simulink model "RendezvousSimulator"  (R2026a)
settings: Solver=ode4  StopTime=7200  FixedStep=0.01
values from neighbouring files (symbols this model uses):
  beta_in = zeros(3,1)    [std_run_docking.m]    (also in std_run_rendezvous.m)
  dt = 0.01    [std_run_docking.m]    (also in std_run_rendezvous.m)
  K = lqr(A,B,Q, R)    [std_run_rendezvous.m]
  muEarth = 3.986004418e14    (= 398600441800000)    [std_run_docking.m]    (also in std_run_rendezvous.m)
  P_in = eye(6) * 1e-4    [std_run_docking.m]    (also in std_run_rendezvous.m)
  q_ic = [1;0;0;0]    [std_run_docking.m]    (also in std_run_rendezvous.m)
  u_ref = -B\(A*xref)    [std_run_rendezvous.m]
  xref = [chaser_CoM_target; 0; 0; 0]    [std_run_docking.m]    (also in std_run_rendezvous.m = [-250, 0, 0, 0.05, 0, 0]')
undefined symbols (not defined in the file or in its folder): ADCS, chaser, control, RCS, RW, target
libraries: aerolibutil x6, simulink x5, simulink_extras x3, matrix_library x1, vrlib x1, mpclib x1, aerolibnav x1
settings Model: SimulationMode=accelerator  Creator=Guilherme  LastModifiedBy=User

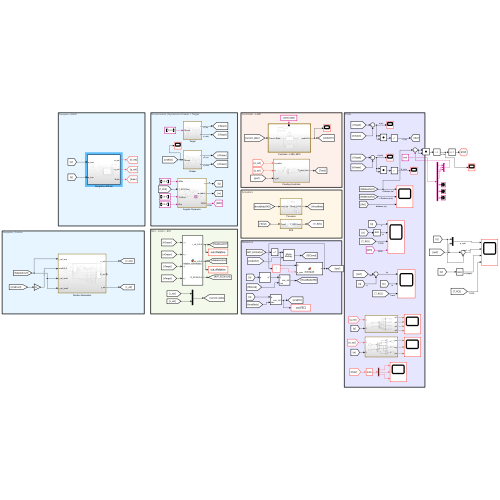
[thumbnail: Simulink's stored preview of the top-level diagram]
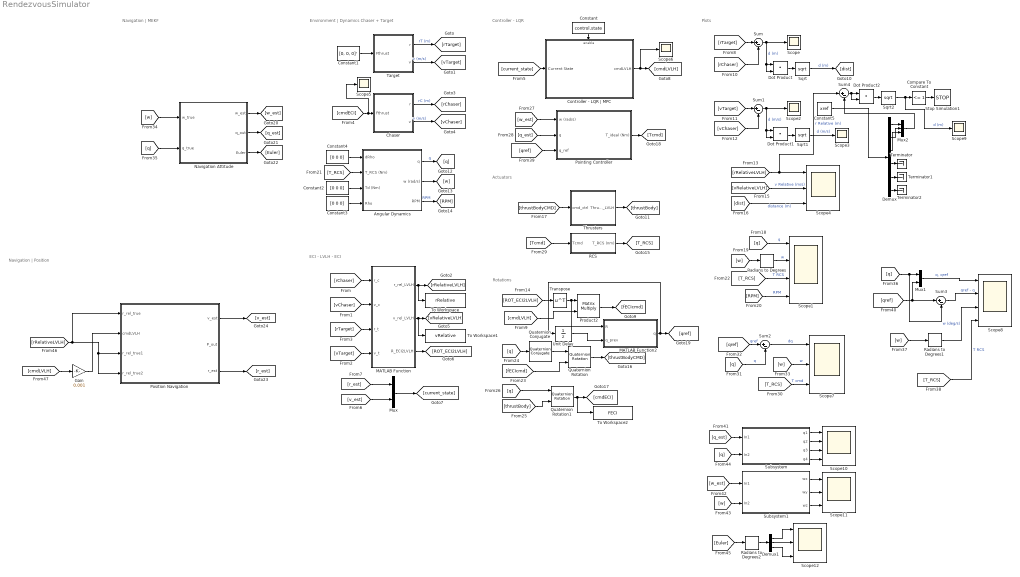
== system RendezvousSimulator ==
  note: Rotations
  note: Actuators
  note: ECI - LVLH - ECI
  note: Controller - LQR
  note: Environment | Dynamics Chaser + Target
  note: Navigation | MEKF
  note: Plots
  note: Navigation | Position
  Angular Dynamics : Subsystem
  Chaser : Subsystem
  Compare To Constant : simulink/Logic and Bit Operations/Compare To Constant  relop=<=  const=1  OutDataTypeStr=boolean
  Constant : Constant  Value=control.state
  Constant1 : Constant  Value=[0, 0, 0]'
  Constant2 : Constant  Value=[0 0 0]
  Constant3 : Constant  Value=[0 0 0]
  Constant4 : Constant  Value=[0 0 0]
  Constant5 : Constant  Value=xref
  Controller - LQR | MPC : Subsystem
  Demux : Demux  Outputs=6
  Demux1 : Demux  Outputs=3
  Dot Product : DotProduct  OutDataTypeStr=Inherit: Inherit via internal rule
  Dot Product1 : DotProduct  OutDataTypeStr=Inherit: Inherit via internal rule
  Dot Product2 : DotProduct  OutDataTypeStr=Inherit: Inherit via internal rule
  Gain : Gain  Gain=0.001
  MATLAB Function : MATLAB Function  TreatAsAtomicUnit=on
  MATLAB Function2 : MATLAB Function  TreatAsAtomicUnit=on
  Mux : Mux  Inputs=2
  Mux1 : Mux  Inputs=2
  Mux2 : Mux  Inputs=3
  Navigation Attitude : Subsystem
  Pointing Controller : Subsystem
  Position Navigation : Subsystem
  Product2 : Product  Multiplication=Matrix(*)
  Quaternion Conjugate : aerolibutil/Quaternion Conjugate
  Quaternion Rotation : aerolibutil/Quaternion Rotation
  Quaternion Rotation1 : aerolibutil/Quaternion Rotation
  RCS : Subsystem
  Radians to Degrees : simulink_extras/Transformations/Radians to Degrees
  Radians to Degrees1 : simulink_extras/Transformations/Radians to Degrees
  Radians to Degrees2 : simulink_extras/Transformations/Radians to Degrees
  Scope{,2..3,5..6,9} (6 alike) : Scope
      Scope settings: ActiveDisplayYMinimum=-1060.8843099508601  ActiveDisplayYMaximum=894.14977464646563
      Scope2 settings: ActiveDisplayYMinimum=-1  ActiveDisplayYMaximum=1  DataLoggingVariableName=ScopeData2
      Scope3 settings: ActiveDisplayYMinimum=-1  ActiveDisplayYMaximum=1  DataLoggingVariableName=ScopeData3
      Scope5 settings: ActiveDisplayYMinimum=-8.2979644162863622  ActiveDisplayYMaximum=33.856564576377387  DataLoggingVariableName=ScopeData5
      Scope6 settings: ActiveDisplayYMinimum=-1  ActiveDisplayYMaximum=1  DataLoggingVariableName=ScopeData6
      Scope9 settings: ActiveDisplayYMinimum=-855.71515275184811  ActiveDisplayYMaximum=7759.3343036097422  DataLoggingVariableName=ScopeData16
  Scope1 : Scope  NumInputPorts=4
      settings: ActiveDisplayYMinimum=-0.12499999999999997  ActiveDisplayYMaximum=1.125  DataLoggingVariableName=ScopeData7
  Scope10 : Scope  NumInputPorts=4
      settings: ActiveDisplayYMinimum=-1  ActiveDisplayYMaximum=1  DataLoggingVariableName=ScopeData17
  Scope{4,7,11..12} (4 alike) : Scope  NumInputPorts=3
      Scope11 settings: ActiveDisplayYMinimum=-0.006211242993111819  ActiveDisplayYMaximum=0.0063918392422366421  DataLoggingVariableName=ScopeData18
      Scope12 settings: ActiveDisplayYMinimum=-0.04294458122283102  ActiveDisplayYMaximum=0.042529284958808582  DataLoggingVariableName=ScopeData19
      Scope4 settings: ActiveDisplayYMinimum=-521.32635380799536  ActiveDisplayYMaximum=173.1359744426077  DataLoggingVariableName=ScopeData4
      Scope7 settings: ActiveDisplayYMinimum=-0.011828379058664178  ActiveDisplayYMaximum=0.0155264540868424  DataLoggingVariableName=ScopeData8
  Scope8 : Scope  NumInputPorts=4
      settings: ActiveDisplayYMinimum=-1.130569243154838  ActiveDisplayYMaximum=1.2367299159060932  DataLoggingVariableName=ScopeData12
  Sqrt : Sqrt
  Sqrt1 : Sqrt
  Sqrt2 : Sqrt
  Stop Simulation1 : Stop
  Subsystem : Subsystem
  Subsystem1 : Subsystem
  Sum{,1..4} (5 alike) : Sum  Inputs=|+-
  Target : Subsystem
  Terminator : Terminator
  Terminator1 : Terminator
  Terminator2 : Terminator
  Thrusters : Subsystem
  To Workspace : ToWorkspace  VariableName=rRelative  SaveFormat=Structure With Time  SampleTime=-1
  To Workspace1 : ToWorkspace  VariableName=vRelative  SaveFormat=Structure With Time  SampleTime=-1
  To Workspace2 : ToWorkspace  VariableName=FECI  SaveFormat=Structure With Time  SampleTime=-1
  Transpose : Math  Operator=transpose
  Unit Delay : UnitDelay  InitialCondition=[1;0;0;0]  SampleTime=dt
  wires:
  Constant1/1 -> Target/1(Fthrust)
  Target/1(r) -> [rTarget]  "rT (m)"
  Target/2(v) -> [vTarget]  "v (m/s)"
  Chaser/1(r) -> [rChaser]  "rC (m)"
  Chaser/2(v) -> [vChaser]  "v (m/s)"
  Mux/1 -> [current_state]
  [r_est] -> Mux/1
  [v_est] -> Mux/2
  Transpose/1 -> MATLAB Function2/1(R), Product2/1
  [ROT_ECI2LVLH] -> Transpose/1
  [cmdLVLH] -> Product2/2
  [cmdECI] -> Scope5/1, Chaser/1(Fthrust)
  [rChaser] -> MATLAB Function/1(r_c)
  [vChaser] -> MATLAB Function/2(v_c)
  [vTarget] -> MATLAB Function/4(v_t)
  [rTarget] -> MATLAB Function/3(r_t)
  MATLAB Function/1(r_rel_LVLH) -> [rRelativeLVLH], To Workspace/1
  MATLAB Function/2(v_rel_LVLH) -> [vRelativeLVLH], To Workspace1/1
  MATLAB Function/3(R_ECI2LVLH) -> [ROT_ECI2LVLH]
  Product2/1 -> [fECIcmd]
  [current_state] -> Controller - LQR | MPC/1(Current State)
  Controller - LQR | MPC/1(cmdLVLH) -> Scope6/1, [cmdLVLH]
  [rTarget] -> Sum/1
  [rChaser] -> Sum/2
  Sum/1 -> Scope/1, Dot Product/2, Dot Product/1  "d (m)"
  Dot Product/1 -> Sqrt/1
  Sqrt/1 -> [dist]  "d (m)"
  Sqrt1/1 -> Scope3/1  "d (m/s)"
  Sum1/1 -> Scope2/1, Dot Product1/2, Dot Product1/1  "d (m/s)"
  Dot Product1/1 -> Sqrt1/1
  [vChaser] -> Sum1/2
  [vTarget] -> Sum1/1
  Compare To Constant/1 -> Stop Simulation1/1
  [rRelativeLVLH] -> Sum4/1, Scope4/1  "r Relative (m)"
  [vRelativeLVLH] -> Scope4/2  "v Relative (m/s)"
  [dist] -> Scope4/3  "distance (m)"
  [thrustBodyCMD] -> Thrusters/1(cmd_ctrl)
  Thrusters/1(Thrust_LVLH) -> [thrustBody]
  Constant/1 -> Controller - LQR | MPC/Enable
  Constant2/1 -> Angular Dynamics/3(Td (Nm))
  Constant3/1 -> Angular Dynamics/4(Rho)
  Constant4/1 -> Angular Dynamics/1(dRho)
  Angular Dynamics/1(q) -> [q]  "q"
  Angular Dynamics/2(w (rad/s)) -> [w]
  Angular Dynamics/3(RPM) -> [RPM]  "RPM"
  [q] -> Scope1/1  "q"
  Radians to Degrees/1 -> Scope1/2  "w"
  [w] -> Radians to Degrees/1
  [RPM] -> Scope1/4  "RPM"
  [Tcmd] -> RCS/1(Tcmd)
  RCS/1(T_RCS (nm)) -> [T_RCS]
  [T_RCS] -> Scope1/3  "T RCS"
  [q] -> Quaternion Conjugate/1
  Quaternion Conjugate/1 -> Quaternion Rotation/1
  [fECIcmd] -> Quaternion Rotation/2
  Quaternion Rotation/1 -> [thrustBodyCMD]
  [thrustBody] -> Quaternion Rotation1/2
  [q] -> Quaternion Rotation1/1
  Quaternion Rotation1/1 -> To Workspace2/1, [cmdECI]
  [w_est] -> Pointing Controller/1(w (rad/s))
  [q_est] -> Pointing Controller/2(q)
  Pointing Controller/1(T_ideal (Nm)) -> [Tcmd]
  MATLAB Function2/1(q) -> Unit Delay/1, [qref]
  [qref] -> Pointing Controller/3(q_ref)
  [w] -> Scope7/2  "w"
  Sum2/1 -> Scope7/1  "dq"
  [q] -> Sum2/2  "q"
  [qref] -> Sum2/1  "qref"
  [T_RCS] -> Scope7/3  "T cmd"
  [q] -> Sum3/2, Mux1/1
  [qref] -> Sum3/1, Mux1/2
  Mux1/1 -> Scope8/1  "q, qref"
  Sum3/1 -> Scope8/2  "qref - q"
  [w] -> Radians to Degrees1/1
  Radians to Degrees1/1 -> Scope8/3  "w (deg/s)"
  [T_RCS] -> Angular Dynamics/2(T_RCS (Nm))
  [T_RCS] -> Scope8/4  "T RCS"
  Sum4/1 -> Dot Product2/2, Dot Product2/1
  Dot Product2/1 -> Sqrt2/1
  Sqrt2/1 -> Scope9/1, Compare To Constant/1  "d (m)"
  Demux/1 -> Mux2/1
  Demux/2 -> Mux2/2
  Demux/3 -> Mux2/3
  Constant5/1 -> Demux/1
  Mux2/1 -> Sum4/2
  Demux/4 -> Terminator/1
  Demux/5 -> Terminator1/1
  Demux/6 -> Terminator2/1
  [w] -> Navigation Attitude/1(w_true)
  [q] -> Navigation Attitude/2(q_true)
  Navigation Attitude/1(w_est) -> [w_est]
  Navigation Attitude/2(q_out) -> [q_est]
  Navigation Attitude/3(Euler) -> [Euler]
  [Euler] -> Radians to Degrees2/1
  Radians to Degrees2/1 -> Demux1/1
  Demux1/1 -> Scope12/1
  Demux1/2 -> Scope12/2
  Demux1/3 -> Scope12/3
  [q_est] -> Subsystem/1(In1)
  [q] -> Subsystem/2(In2)
  Subsystem/1(q1) -> Scope10/1
  Subsystem/2(q2) -> Scope10/2
  Subsystem/3(q3) -> Scope10/3
  Subsystem/4(q4) -> Scope10/4
  [w] -> Subsystem1/2(In2)
  Subsystem1/1(wx) -> Scope11/1
  Subsystem1/2(wy) -> Scope11/2
  Subsystem1/3(wz) -> Scope11/3
  [w_est] -> Subsystem1/1(In1)
  Unit Delay/1 -> MATLAB Function2/2(q_prev)
  Position Navigation/3(r_est) -> [r_est]
  Gain/1 -> Position Navigation/2(cmdLVLH)
  [cmdLVLH] -> Gain/1
  Position Navigation/1(v_est) -> [v_est]
  [rRelativeLVLH] -> Position Navigation/4(r_rel_true2), Position Navigation/3(r_rel_true1), Position Navigation/1(r_rel_true)

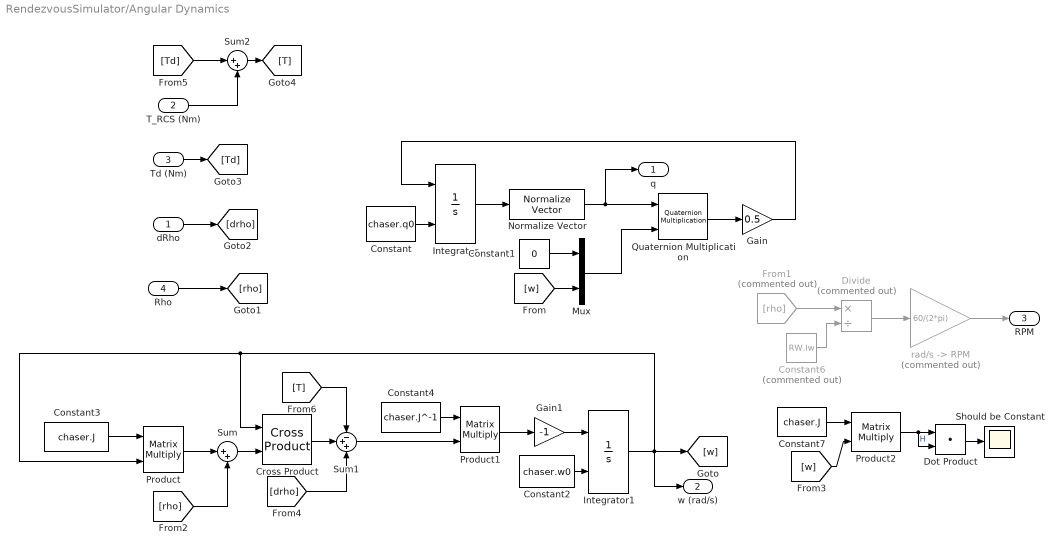
== system RendezvousSimulator/Angular Dynamics ==
  dRho : Inport
  T_RCS (Nm) : Inport  Port=2
  Td (Nm) : Inport  Port=3
  Rho : Inport  Port=4
  Constant : Constant  Value=chaser.q0
  Constant1 : Constant  Value=0
  Constant2 : Constant  Value=chaser.w0
  Constant3 : Constant  Value=chaser.J
  Constant4 : Constant  Value=chaser.J^-1
  Constant6 : Constant  Commented=on  Value=RW.Iw
  Constant7 : Constant  Value=chaser.J
  Cross Product : matrix_library/Cross Product
  Divide : Product  Commented=on  Inputs=*/
  Dot Product : DotProduct  OutDataTypeStr=Inherit: Inherit via internal rule
  From1 : From  Commented=on  GotoTag=rho
  Gain : Gain  Gain=0.5
  Gain1 : Gain  Gain=-1
  Integrator : Integrator  InitialConditionSource=external
  Integrator1 : Integrator  InitialConditionSource=external
  Mux : Mux  Inputs=2
  Normalize Vector : vrlib/Utilities/Normalize Vector  maxzero=0
  Product : Product  Multiplication=Matrix(*)
  Product1 : Product  Multiplication=Matrix(*)
  Product2 : Product  Multiplication=Matrix(*)
  Quaternion Multiplication : aerolibutil/Quaternion Multiplication
  Should be Constant : Scope
      settings: ActiveDisplayYMinimum=4.5666666666666505E-5  ActiveDisplayYMaximum=6.566666666666693E-5
  Sum : Sum  Inputs=|++
  Sum1 : Sum  Inputs=-++
  Sum2 : Sum  Inputs=|++
  "rad/s -> RPM" : Gain  Commented=on  Gain=60/(2*pi)
  q : Outport
  w (rad/s) : Outport  Port=2
  RPM : Outport  Port=3
  wires:
  Normalize Vector/1 -> q/1, Quaternion Multiplication/1
  Quaternion Multiplication/1 -> Gain/1
  Integrator1/1 -> w (rad/s)/1, Product/2, Cross Product/1, [w]
  Constant/1 -> Integrator/2
  Constant2/1 -> Integrator1/2
  [rho] -> Sum/2
  Product1/1 -> Gain1/1
  Gain/1 -> Integrator/1
  Sum/1 -> Cross Product/2
  Constant4/1 -> Product1/1
  Integrator/1 -> Normalize Vector/1
  Sum1/1 -> Product1/2
  Constant1/1 -> Mux/1
  Mux/1 -> Quaternion Multiplication/2
  Product/1 -> Sum/1
  Cross Product/1 -> Sum1/2
  [w] -> Mux/2
  [T] -> Sum1/1
  Gain1/1 -> Integrator1/1
  Constant3/1 -> Product/1
  From1/1 -> Divide/1
  Constant6/1 -> Divide/2
  Divide/1 -> "rad/s -> RPM"/1
  "rad/s -> RPM"/1 -> RPM/1
  Constant7/1 -> Product2/1
  Dot Product/1 -> Should be Constant/1
  Product2/1 -> Dot Product/2, Dot Product/1  "H"
  [w] -> Product2/2
  Td (Nm)/1 -> [Td]
  [Td] -> Sum2/1
  T_RCS (Nm)/1 -> Sum2/2
  Sum2/1 -> [T]
  [drho] -> Sum1/3
  Rho/1 -> [rho]
  dRho/1 -> [drho]

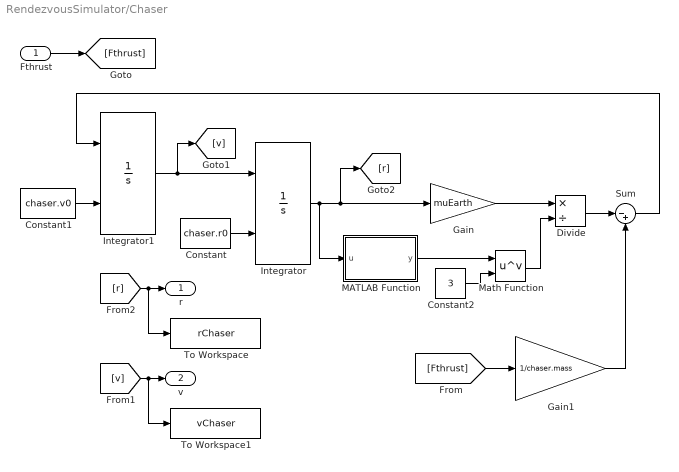
== system RendezvousSimulator/Chaser ==
  Fthrust : Inport
  Constant : Constant  Value=chaser.r0
  Constant1 : Constant  Value=chaser.v0
  Constant2 : Constant  Value=3
  Divide : Product  Inputs=*/
  Gain : Gain  Gain=muEarth
  Gain1 : Gain  Gain=1/chaser.mass
  Integrator : Integrator  InitialConditionSource=external
  Integrator1 : Integrator  InitialConditionSource=external
  MATLAB Function : MATLAB Function  TreatAsAtomicUnit=on
  Math Function : Math  Operator=pow
  Sum : Sum  Inputs=|-+
  To Workspace : ToWorkspace  VariableName=rChaser  SaveFormat=Structure With Time  SampleTime=-1
  To Workspace1 : ToWorkspace  VariableName=vChaser  SaveFormat=Structure With Time  SampleTime=-1
  r : Outport
  v : Outport  Port=2
  wires:
  Integrator/1 -> MATLAB Function/1(u), [r], Gain/1
  Constant1/1 -> Integrator1/2
  Gain/1 -> Divide/1
  Divide/1 -> Sum/1
  Constant/1 -> Integrator/2
  Sum/1 -> Integrator1/1
  Integrator1/1 -> Integrator/1, [v]
  Fthrust/1 -> [Fthrust]
  [Fthrust] -> Gain1/1
  Gain1/1 -> Sum/2
  [v] -> To Workspace1/1, v/1
  [r] -> To Workspace/1, r/1
  MATLAB Function/1(y) -> Math Function/1
  Constant2/1 -> Math Function/2
  Math Function/1 -> Divide/2

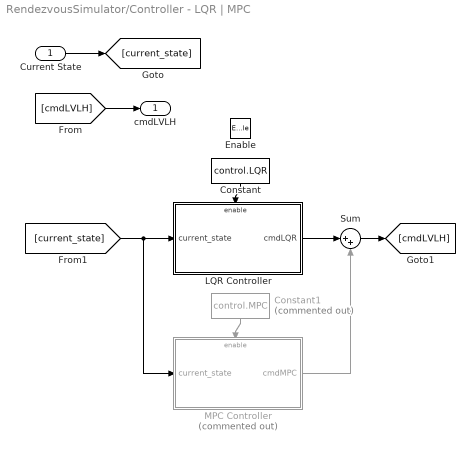
== system RendezvousSimulator/Controller - LQR | MPC ==
  Current State : Inport
  Enable : EnablePort
  Constant : Constant  Value=control.LQR
  Constant1 : Constant  Commented=on  Value=control.MPC
  LQR Controller : Subsystem
  MPC Controller : Subsystem  Commented=on
  Sum : Sum  Inputs=|++
  cmdLVLH : Outport
  wires:
  Current State/1 -> [current_state]
  [cmdLVLH] -> cmdLVLH/1
  Constant/1 -> LQR Controller/Enable
  Constant1/1 -> MPC Controller/Enable
  LQR Controller/1(cmdLQR) -> Sum/1
  MPC Controller/1(cmdMPC) -> Sum/2
  Sum/1 -> [cmdLVLH]
  [current_state] -> MPC Controller/1(current_state), LQR Controller/1(current_state)

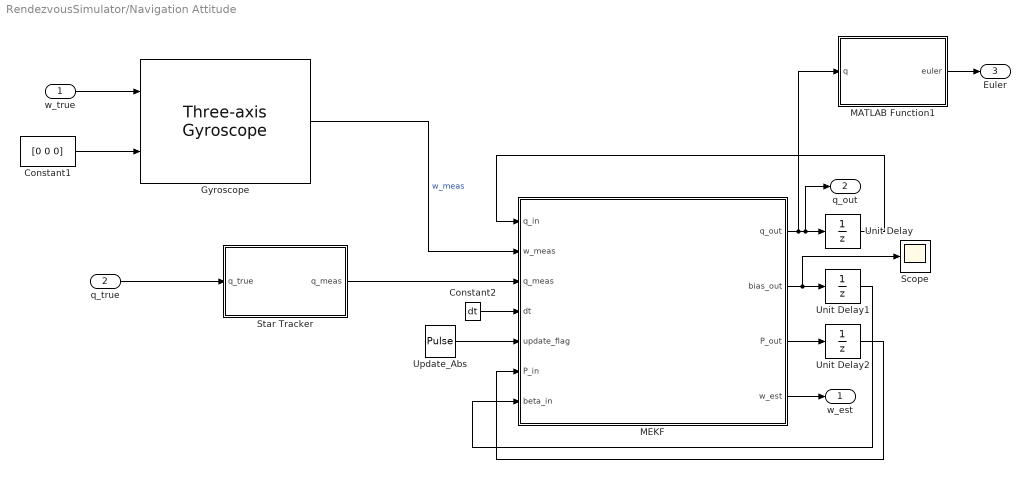
== system RendezvousSimulator/Navigation Attitude ==
  w_true : Inport
  q_true : Inport  Port=2
  Constant1 : Constant  Value=[0 0 0]
  Constant2 : Constant  Value=dt
  Gyroscope : aerolibnav/Three-axis Gyroscope  dtype_g=on  w_g=190  z_g=0.707  g_sf_cc=[1 0 0; 0 1 0; 0 0 1]  g_bias=bias  g_sen=[0 0 0]  g_Ts=dt  g_rand=on  g_seeds=[23093 23094 23095]  g_pow=[1e-8 1e-8 1e-8]  g_sat="[-inf  -inf  -inf  inf inf inf]"
  MATLAB Function1 : MATLAB Function  TreatAsAtomicUnit=on
  MEKF : MATLAB Function  TreatAsAtomicUnit=on  SystemSampleTime=dt
  Scope : Scope
      settings: ActiveDisplayYMinimum=-0.0039936998419851629  ActiveDisplayYMaximum=0.0043770375414137726  DataLoggingVariableName=ScopeData20
  Star Tracker : MATLAB Function  TreatAsAtomicUnit=on
  Unit Delay : UnitDelay  InitialCondition=q_ic  SampleTime=dt
  Unit Delay1 : UnitDelay  InitialCondition=beta_in  SampleTime=dt
  Unit Delay2 : UnitDelay  InitialCondition=P_in  SampleTime=dt
  Update_Abs : DiscretePulseGenerator  Period=100  SampleTime=dt
  w_est : Outport
  q_out : Outport  Port=2
  Euler : Outport  Port=3
  wires:
  Constant2/1 -> MEKF/4(dt)
  Unit Delay/1 -> MEKF/1(q_in)
  MEKF/4(w_est) -> w_est/1
  Unit Delay1/1 -> MEKF/7(beta_in)
  Unit Delay2/1 -> MEKF/6(P_in)
  MEKF/2(bias_out) -> Scope/1, Unit Delay1/1
  Constant1/1 -> Gyroscope/2
  MEKF/3(P_out) -> Unit Delay2/1
  MEKF/1(q_out) -> Unit Delay/1, q_out/1, MATLAB Function1/1(q)
  w_true/1 -> Gyroscope/1
  q_true/1 -> Star Tracker/1(q_true)
  Star Tracker/1(q_meas) -> MEKF/3(q_meas)
  Gyroscope/1 -> MEKF/2(w_meas)  "w_meas"
  Update_Abs/1 -> MEKF/5(update_flag)
  MATLAB Function1/1(euler) -> Euler/1

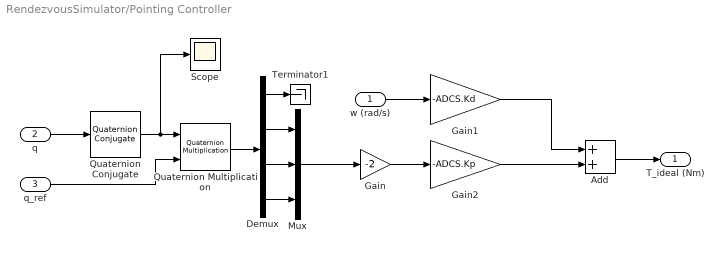
== system RendezvousSimulator/Pointing Controller ==
  w (rad/s) : Inport
  q : Inport  Port=2
  q_ref : Inport  Port=3
  Add : Sum
  Demux : Demux
  Gain : Gain  Gain=-2
  Gain1 : Gain  Gain=-ADCS.Kd
  Gain2 : Gain  Gain=-ADCS.Kp
  Mux : Mux  Inputs=3
  Quaternion Conjugate : aerolibutil/Quaternion Conjugate
  Quaternion Multiplication : aerolibutil/Quaternion Multiplication
  Scope : Scope
      settings: ActiveDisplayYMinimum=-1  ActiveDisplayYMaximum=1  DataLoggingVariableName=ScopeData6
  Terminator1 : Terminator
  T_ideal (Nm) : Outport
  wires:
  Mux/1 -> Gain/1
  Quaternion Conjugate/1 -> Scope/1, Quaternion Multiplication/1
  Gain2/1 -> Add/2
  Demux/3 -> Mux/2
  Gain/1 -> Gain2/1
  q_ref/1 -> Quaternion Multiplication/2
  Demux/2 -> Mux/1
  q/1 -> Quaternion Conjugate/1
  w (rad/s)/1 -> Gain1/1
  Demux/4 -> Mux/3
  Demux/1 -> Terminator1/1
  Gain1/1 -> Add/1
  Quaternion Multiplication/1 -> Demux/1
  Add/1 -> T_ideal (Nm)/1

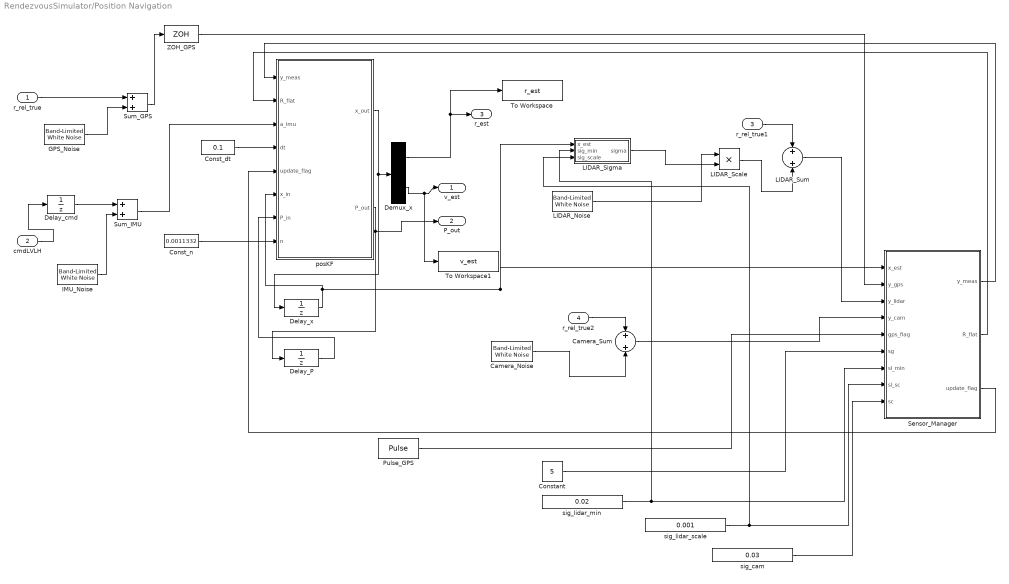
== system RendezvousSimulator/Position Navigation ==
  r_rel_true : Inport
  cmdLVLH : Inport  Port=2
  r_rel_true1 : Inport  Port=3
  r_rel_true2 : Inport  Port=4
  Camera_Noise : simulink/Sources/Band-Limited White Noise  Cov=[9e-05; 9e-05; 9e-05]  Ts=0.1  seed=[23341]
  Camera_Sum : Sum
  Const_dt : Constant  Value=0.1  SampleTime=0.1
  Const_n : Constant  Value=0.0011332  SampleTime=0.1
  Constant : Constant  Value=5
  Delay_P : UnitDelay  InitialCondition=[2500 0 0 0 0 0;0 2500 0 0 0 0;0 0 2500 0 0 0;0 0 0 25 0 0;0 0 0 0 25 0;0 0 0 0 0 25]  SampleTime=0.1
  Delay_cmd : UnitDelay  InitialCondition=[0;0;0]  SampleTime=0.1
  Delay_x : UnitDelay  InitialCondition=[-250;0;0;0;0;0]  SampleTime=0.1
  Demux_x : Demux  Outputs=[3 3]
  GPS_Noise : simulink/Sources/Band-Limited White Noise  Cov=[25 25 25]  Ts=1  seed=[23341 23342 23343]
  IMU_Noise : simulink/Sources/Band-Limited White Noise  Cov=[1e-05 1e-05 1e-05]  Ts=0.1  seed=[12341 12342 12343]
  LIDAR_Noise : simulink/Sources/Band-Limited White Noise  Cov=[0.1; 0.1; 0.1]  Ts=0.1  seed=[23341]
  LIDAR_Scale : Product  Inputs=**
  LIDAR_Sigma : MATLAB Function  TreatAsAtomicUnit=on
  LIDAR_Sum : Sum
  Pulse_GPS : DiscretePulseGenerator  PulseType=Time based  Period=1  PulseWidth=10  SampleTime=0.1
  Sensor_Manager : MATLAB Function  TreatAsAtomicUnit=on
  Sum_GPS : Sum
  Sum_IMU : Sum
  To Workspace : ToWorkspace  VariableName=r_est  SaveFormat=Structure With Time  SampleTime=-1
  To Workspace1 : ToWorkspace  VariableName=v_est  SaveFormat=Structure With Time  SampleTime=-1
  ZOH_GPS : ZeroOrderHold
  posKF : MATLAB Function  TreatAsAtomicUnit=on
  sig_cam : Constant  Value=0.03
  sig_lidar_min : Constant  Value=0.02
  sig_lidar_scale : Constant  Value=0.001
  v_est : Outport
  P_out : Outport  Port=2
  r_est : Outport  Port=3
  wires:
  r_rel_true/1 -> Sum_GPS/1
  GPS_Noise/1 -> Sum_GPS/2
  Sum_GPS/1 -> ZOH_GPS/1
  Pulse_GPS/1 -> Sensor_Manager/5(gps_flag)
  cmdLVLH/1 -> Delay_cmd/1
  Delay_cmd/1 -> Sum_IMU/1
  IMU_Noise/1 -> Sum_IMU/2
  Sum_IMU/1 -> posKF/3(a_imu)
  Const_dt/1 -> posKF/4(dt)
  Const_n/1 -> posKF/8(n)
  Delay_x/1 -> Sensor_Manager/1(x_est), LIDAR_Sigma/1(x_est), posKF/6(x_in)
  Delay_P/1 -> posKF/7(P_in)
  posKF/1(x_out) -> Delay_x/1, Demux_x/1
  posKF/2(P_out) -> Delay_P/1, P_out/1
  Demux_x/1 -> To Workspace/1, r_est/1
  Demux_x/2 -> To Workspace1/1, v_est/1
  LIDAR_Noise/1 -> LIDAR_Scale/1
  LIDAR_Sigma/1(sigma) -> LIDAR_Scale/2
  LIDAR_Scale/1 -> LIDAR_Sum/2
  Camera_Noise/1 -> Camera_Sum/2
  sig_lidar_min/1 -> LIDAR_Sigma/2(sig_min), Sensor_Manager/7(sl_min)
  sig_lidar_scale/1 -> LIDAR_Sigma/3(sig_scale), Sensor_Manager/8(sl_sc)
  sig_cam/1 -> Sensor_Manager/9(sc)
  r_rel_true1/1 -> LIDAR_Sum/1
  r_rel_true2/1 -> Camera_Sum/1
  LIDAR_Sum/1 -> Sensor_Manager/3(y_lidar)
  Camera_Sum/1 -> Sensor_Manager/4(y_cam)
  ZOH_GPS/1 -> Sensor_Manager/2(y_gps)
  Constant/1 -> Sensor_Manager/6(sg)
  Sensor_Manager/3(update_flag) -> posKF/5(update_flag)
  Sensor_Manager/1(y_meas) -> posKF/1(y_meas)
  Sensor_Manager/2(R_flat) -> posKF/2(R_flat)

== system RendezvousSimulator/RCS ==
  Tcmd : Inport
  Manual Switch : ManualSwitch
  PWM RCS : Subsystem
  Simple RCS : Subsystem
  T_RCS (nm) : Outport
  wires:
  Tcmd/1 -> PWM RCS/1(Tcmd), Simple RCS/1(Tcmd)
  Simple RCS/1(Treal) -> Manual Switch/1
  PWM RCS/1(Treal) -> Manual Switch/2
  Manual Switch/1 -> T_RCS (nm)/1

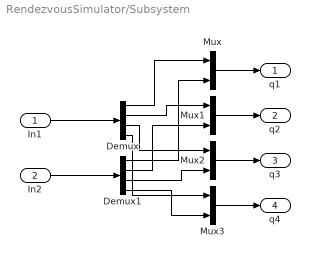
== system RendezvousSimulator/Subsystem ==
  In1 : Inport
  In2 : Inport  Port=2
  Demux : Demux
  Demux1 : Demux
  Mux{,1..3} (4 alike) : Mux  Inputs=2
  q1 : Outport
  q2 : Outport  Port=2
  q3 : Outport  Port=3
  q4 : Outport  Port=4
  wires:
  In2/1 -> Demux1/1
  In1/1 -> Demux/1
  Demux/1 -> Mux/1
  Demux1/1 -> Mux/2
  Demux/2 -> Mux1/1
  Demux1/2 -> Mux1/2
  Demux/3 -> Mux2/1
  Demux1/3 -> Mux2/2
  Demux/4 -> Mux3/1
  Demux1/4 -> Mux3/2
  Mux/1 -> q1/1
  Mux1/1 -> q2/1
  Mux2/1 -> q3/1
  Mux3/1 -> q4/1

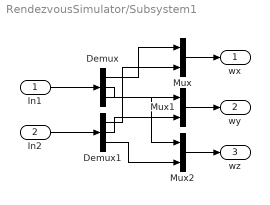
== system RendezvousSimulator/Subsystem1 ==
  In1 : Inport
  In2 : Inport  Port=2
  Demux : Demux  Outputs=3
  Demux1 : Demux  Outputs=3
  Mux : Mux  Inputs=2
  Mux1 : Mux  Inputs=2
  Mux2 : Mux  Inputs=2
  wx : Outport
  wy : Outport  Port=2
  wz : Outport  Port=3
  wires:
  In1/1 -> Demux/1
  In2/1 -> Demux1/1
  Demux/1 -> Mux/1
  Demux1/1 -> Mux/2
  Demux/2 -> Mux1/1
  Demux1/2 -> Mux1/2
  Demux/3 -> Mux2/1
  Demux1/3 -> Mux2/2
  Mux2/1 -> wz/1
  Mux1/1 -> wy/1
  Mux/1 -> wx/1

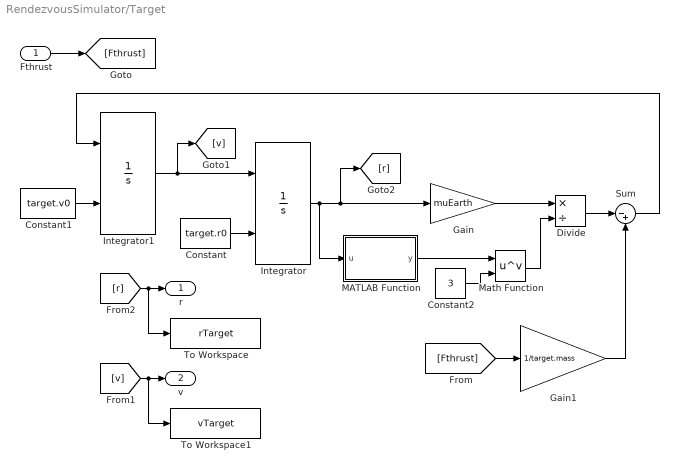
== system RendezvousSimulator/Target ==
  Fthrust : Inport
  Constant : Constant  Value=target.r0
  Constant1 : Constant  Value=target.v0
  Constant2 : Constant  Value=3
  Divide : Product  Inputs=*/
  Gain : Gain  Gain=muEarth
  Gain1 : Gain  Gain=1/target.mass
  Integrator : Integrator  InitialConditionSource=external
  Integrator1 : Integrator  InitialConditionSource=external
  MATLAB Function : MATLAB Function  TreatAsAtomicUnit=on
  Math Function : Math  Operator=pow
  Sum : Sum  Inputs=|-+
  To Workspace : ToWorkspace  VariableName=rTarget  SaveFormat=Structure With Time  SampleTime=-1
  To Workspace1 : ToWorkspace  VariableName=vTarget  SaveFormat=Structure With Time  SampleTime=-1
  r : Outport
  v : Outport  Port=2
  wires:
  Math Function/1 -> Divide/2
  Constant2/1 -> Math Function/2
  MATLAB Function/1(y) -> Math Function/1
  [r] -> r/1, To Workspace/1
  [v] -> v/1, To Workspace1/1
  Gain1/1 -> Sum/2
  [Fthrust] -> Gain1/1
  Fthrust/1 -> [Fthrust]
  Integrator1/1 -> [v], Integrator/1
  Sum/1 -> Integrator1/1
  Constant/1 -> Integrator/2
  Divide/1 -> Sum/1
  Gain/1 -> Divide/1
  Constant1/1 -> Integrator1/2
  Integrator/1 -> Gain/1, [r], MATLAB Function/1(u)

== system RendezvousSimulator/Thrusters ==
  cmd_ctrl : Inport
  Gain : Gain  Commented=on  Gain=50
  Saturation : Saturate  UpperLimit=50*[1, 1, 1]'  LowerLimit=-50*[1, 1, 1]'
  Scope : Scope
      settings: ActiveDisplayYMinimum=-54.314607506829162  ActiveDisplayYMaximum=51.882871006307695
  Sign : Signum  Commented=on
  Thrust_LVLH : Outport
  wires:
  cmd_ctrl/1 -> Saturation/1
  Saturation/1 -> Scope/1, Thrust_LVLH/1
  Sign/1 -> Gain/1

== system RendezvousSimulator/Controller - LQR | MPC/LQR Controller ==
  current_state : Inport
  Enable : EnablePort
  Constant : Constant  Value=xref
  Constant1 : Constant  Value=u_ref
  Gain : Gain  Gain=K  Multiplication=Matrix(K*u)
  Sum : Sum  Inputs=|+-
  Sum1 : Sum  Inputs=|++
  cmdLQR : Outport
  wires:
  current_state/1 -> Sum/2
  Constant/1 -> Sum/1
  Sum/1 -> Gain/1
  Sum1/1 -> cmdLQR/1
  Gain/1 -> Sum1/1
  Constant1/1 -> Sum1/2

== system RendezvousSimulator/Controller - LQR | MPC/MPC Controller ==
  current_state : Inport
  Enable : EnablePort
  Constant : Constant  Value=xref
  MPC Controller : mpclib/MPC Controller  SCDEnableBlockLinearizationSpecification=on  mpcobj=mpc_controller  is_multiple=0  enable_value=0  return_u0=off  updateMPCinCallerWorkspace=on  md_inport=off  mv_inport=off  uref_inport=off  return_cost=off  return_mvseq=off  return_qpstatus=off  return_xseq=off  return_state=off  return_ovseq=off  state_inport=off  umin_inport=off  umax_inport=off  ymin_inport=off  ymax_inport=off  cc_inport=off  ywt_inport=off  uwt_inport=off  duwt_inport=off  rhoeps_inport=off  pm_inport=off  MaximumP=10  HorizonChoice=FixedHorizon  n_ts=1  n_p=50  n_mv=3  n_md=0  n_ud=0  n_mo=6  n_uo=0  BlockDataType=double  SampleTimeInherited=off  switch_inport=off
  cmdMPC : Outport
  wires:
  MPC Controller/1 -> cmdMPC/1
  current_state/1 -> MPC Controller/1
  Constant/1 -> MPC Controller/2

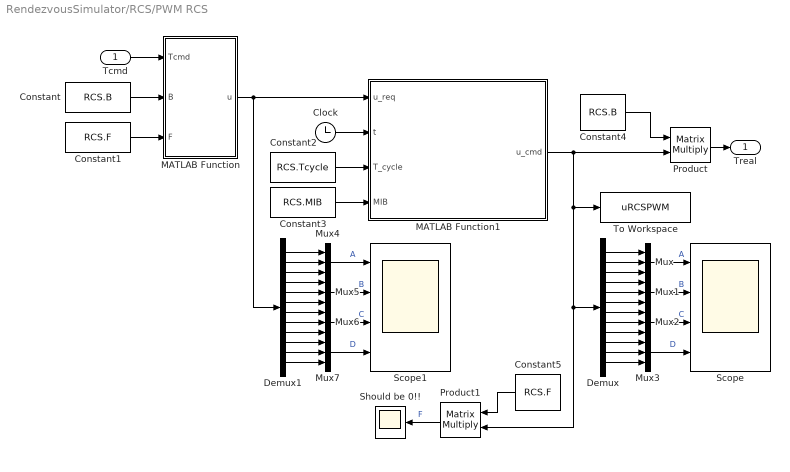
== system RendezvousSimulator/RCS/PWM RCS ==
  Tcmd : Inport
  Clock : Clock
  Constant : Constant  Value=RCS.B
  Constant1 : Constant  Value=RCS.F
  Constant2 : Constant  Value=RCS.Tcycle
  Constant3 : Constant  Value=RCS.MIB
  Constant4 : Constant  Value=RCS.B
  Constant5 : Constant  Value=RCS.F
  Demux : Demux  Outputs=12
  Demux1 : Demux  Outputs=12
  MATLAB Function : MATLAB Function  TreatAsAtomicUnit=on
  MATLAB Function1 : MATLAB Function  TreatAsAtomicUnit=on
  Mux{,1..7} (8 alike) : Mux  Inputs=3
  Product : Product  Multiplication=Matrix(*)
  Product1 : Product  Multiplication=Matrix(*)
  Scope : Scope  NumInputPorts=4
      settings: ActiveDisplayYMinimum=-1  ActiveDisplayYMaximum=1  DataLoggingVariableName=ScopeData13
  Scope1 : Scope  NumInputPorts=4
      settings: ActiveDisplayYMinimum=-1  ActiveDisplayYMaximum=1  DataLoggingVariableName=ScopeData14
  Should be 0!! : Scope
      settings: ActiveDisplayYMinimum=-1  ActiveDisplayYMaximum=1  DataLoggingVariableName=ScopeData15
  To Workspace : ToWorkspace  VariableName=uRCSPWM  SaveFormat=Timeseries  SampleTime=-1
  Treal : Outport
  wires:
  Constant/1 -> MATLAB Function/2(B)
  Constant3/1 -> MATLAB Function1/4(MIB)
  Constant2/1 -> MATLAB Function1/3(T_cycle)
  Constant1/1 -> MATLAB Function/3(F)
  Clock/1 -> MATLAB Function1/2(t)
  Constant4/1 -> Product/1
  Product/1 -> Treal/1
  Tcmd/1 -> MATLAB Function/1(Tcmd)
  Demux/1 -> Mux/1
  Demux/2 -> Mux/2
  Demux/3 -> Mux/3
  Demux/4 -> Mux1/1
  Demux/5 -> Mux1/2
  Demux/6 -> Mux1/3
  Demux/7 -> Mux2/1
  Demux/8 -> Mux2/2
  Demux/9 -> Mux2/3
  Demux/10 -> Mux3/1
  Demux/11 -> Mux3/2
  Demux/12 -> Mux3/3
  Mux/1 -> Scope/1  "A"
  Mux1/1 -> Scope/2  "B"
  Mux2/1 -> Scope/3  "C"
  Mux3/1 -> Scope/4  "D"
  MATLAB Function/1(u) -> Demux1/1, MATLAB Function1/1(u_req)
  Demux1/5 -> Mux5/2
  Mux4/1 -> Scope1/1  "A"
  Mux5/1 -> Scope1/2  "B"
  Demux1/6 -> Mux5/3
  Demux1/4 -> Mux5/1
  Demux1/8 -> Mux6/2
  Demux1/11 -> Mux7/2
  Mux7/1 -> Scope1/4  "D"
  Demux1/7 -> Mux6/1
  Demux1/10 -> Mux7/1
  Mux6/1 -> Scope1/3  "C"
  Demux1/3 -> Mux4/3
  Demux1/9 -> Mux6/3
  Demux1/2 -> Mux4/2
  Demux1/1 -> Mux4/1
  Demux1/12 -> Mux7/3
  Product1/1 -> Should be 0!!/1  "F"
  MATLAB Function1/1(u_cmd) -> Demux/1, Product1/2, To Workspace/1, Product/2
  Constant5/1 -> Product1/1

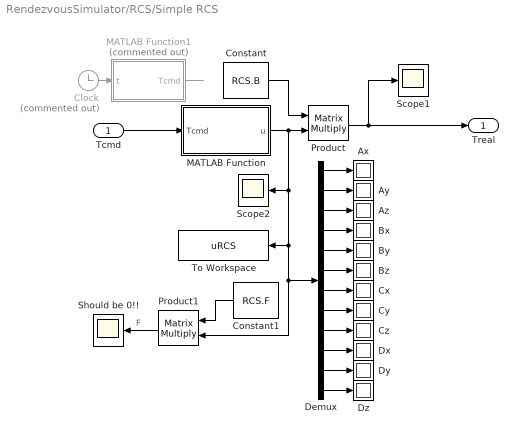
== system RendezvousSimulator/RCS/Simple RCS ==
  Tcmd : Inport
  Ax : Display
  Ay : Display
  Az : Display
  Bx : Display
  By : Display
  Bz : Display
  Clock : Clock  Commented=on
  Constant : Constant  Value=RCS.B
  Constant1 : Constant  Value=RCS.F
  Cx : Display
  Cy : Display
  Cz : Display
  Demux : Demux  Outputs=12
  Dx : Display
  Dy : Display
  Dz : Display
  MATLAB Function : MATLAB Function  TreatAsAtomicUnit=on
  MATLAB Function1 : MATLAB Function  Commented=on  TreatAsAtomicUnit=on
  Product : Product  Multiplication=Matrix(*)
  Product1 : Product  Multiplication=Matrix(*)
  Scope1 : Scope
      settings: ActiveDisplayYMinimum=-0.31914893617021267  ActiveDisplayYMaximum=0.13677811550151975  DataLoggingVariableName=ScopeData9
  Scope2 : Scope
      settings: ActiveDisplayYMinimum=-0.056610942249240015  ActiveDisplayYMaximum=1.0224164133738602  DataLoggingVariableName=ScopeData10
  Should be 0!! : Scope
      settings: ActiveDisplayYMinimum=-1  ActiveDisplayYMaximum=1  DataLoggingVariableName=ScopeData11
  To Workspace : ToWorkspace  VariableName=uRCS  SaveFormat=Timeseries  SampleTime=-1
  Treal : Outport
  wires:
  Demux/11 -> Dy/1
  MATLAB Function/1(u) -> To Workspace/1, Product1/2, Demux/1, Scope2/1, Product/2
  Demux/2 -> Ay/1
  Demux/8 -> Cy/1
  Demux/6 -> Bz/1
  Product/1 -> Treal/1, Scope1/1
  Demux/10 -> Dx/1
  Constant1/1 -> Product1/1
  Constant/1 -> Product/1
  Demux/3 -> Az/1
  Product1/1 -> Should be 0!!/1  "F"
  Demux/1 -> Ax/1
  Clock/1 -> MATLAB Function1/1(t)
  Demux/12 -> Dz/1
  Demux/9 -> Cz/1
  Demux/5 -> By/1
  Demux/4 -> Bx/1
  Demux/7 -> Cx/1
  Tcmd/1 -> MATLAB Function/1(Tcmd)
  MATLAB Function1/1(Tcmd) -> ?

== matlab function RendezvousSimulator/Navigation Attitude/MATLAB Function1 ==
  data: q input; euler output
function euler = quat2euler(q)
    % Convert quaternion to Euler angles (roll, pitch, yaw)
    % Input:  q = [qw, qx, qy, qz] (normalized quaternion)
    % Output: euler = [roll, pitch, yaw] in radians (ZYX convention)
    
    % Normalize the quaternion (safety check)
    q = q / norm(q);
    qw = q(1); qx = q(2); qy = q(3); qz = q(4);
    
    % Roll (rotation about X axis)
    roll  = atan2(2*(qw*qx + qy*qz), 1 - 2*(qx^2 + qy^2));
    
    % Pitch (rotation about Y axis) - with gimbal lock protection
    sinp = 2*(qw*qy - qz*qx);
    if abs(sinp) >= 1
        pitch = sign(sinp) * pi/2;  % clamp to ±90° at gimbal lock
    else
        pitch = asin(sinp);
    end
    
    % Yaw (rotation about Z axis)
    yaw   = atan2(2*(qw*qz + qx*qy), 1 - 2*(qy^2 + qz^2));
    
    euler = [roll, pitch, yaw];
end

== matlab function RendezvousSimulator/Navigation Attitude/MEKF ==
  settings: updateMethod=DISCRETE  sampleTime=0.01
  data: q_in input size=[4 1]; w_meas input; q_out output; q_meas input size=[4 1]; dt input; update_flag input; bias_out output; P_in input; beta_in input; P_out output; w_est output
function [q_out, bias_out, P_out, w_est] = fcn(q_in, w_meas, q_meas, dt, update_flag, P_in, beta_in)
% MULTIPLICATIVE EXTENDED KALMAN FILTER (MEKF) — Robust Sequential Update
% Convention: Hamiltonian, Unit Quaternion, Scalar-First [w; x; y; z]
% =========================================================================
% 1. INPUT NORMALIZATION (With divide-by-zero protection)
% =========================================================================
q_in       = q_in(:)       / (norm(q_in) + 1e-12);
q_meas     = q_meas(:)     / (norm(q_meas) + 1e-12);
w_meas     = w_meas(:);
beta_est   = beta_in(:);
P          = P_in;

% =========================================================================
% 2. TUNING PARAMETERS
% =========================================================================
Q_noise = diag([1e-5, 1e-5, 1e-5, 1e-10, 1e-10, 1e-10]);
R_total = eye(3) * (9.7e-5)^2;   % Star tracker accuracy ~20 arcsec

% =========================================================================
% PHASE 1 — PREDICTION (TIME UPDATE)
% =========================================================================
w_hat   = w_meas - beta_est;
mag_w   = norm(w_hat);
if mag_w > 1e-12
    dq_prop = [cos(0.5 * mag_w * dt); (w_hat / mag_w) * sin(0.5 * mag_w * dt)];
else
    dq_prop = [1; 0; 0; 0];
end

% Propagate quaternion using the safe local function
q_minus = quat_mult(q_in, dq_prop);

% Propagate state covariance matrix
W_skew = [       0,   -w_hat(3),  w_hat(2);
           w_hat(3),        0,   -w_hat(1);
          -w_hat(2),  w_hat(1),        0  ];
          
Phi = [eye(3) - W_skew*dt,  -eye(3)*dt;
       zeros(3,3),            eye(3)   ];
       
P = Phi * P * Phi' + Q_noise * dt;

% Enforce symmetry to prevent numerical drift anomalies
P = 0.5 * (P + P'); 

% =========================================================================
% PHASE 2 — CORRECTION (MEASUREMENT UPDATE VIA SEQUENTIAL FILTERING)
% =========================================================================
% Initialize the updated state estimates with the predicted values
q_upd    = q_minus;
beta_upd = beta_est;

% ---- Update 1: Star Tracker (Absolute Attitude) -------------------------
if update_flag > 0.5
    q_upd_inv = [q_upd(1); -q_upd(2:4)];
    q_err = quat_mult(q_upd_inv, q_meas);
    
    % Shortest path constraint (quaternion switching prevention)
    if q_err(1) < 0
        q_err = -q_err;
    end
    
    res = 2 * q_err(2:4);
    H   = [eye(3), zeros(3,3)];

    
    S   = H * P * H' + R_total;
    K   = (P * H') / S;
    dx  = K * res;
    
    % Covariance Update using the numerically stable Joseph Form
    I_KH = eye(6) - K * H;
    P    = I_KH * P * I_KH' + K * R_total * K';
    P    = 0.5 * (P + P'); % Maintain matrix symmetry
    
    % Intermediate Reset (updates q_upd and beta_upd for the next sensor)
    d_theta = dx(1:3);
    mag_dtheta = norm(d_theta);
    if mag_dtheta > 1e-12
        dq_update = [cos(mag_dtheta/2); (d_theta/mag_dtheta)*sin(mag_dtheta/2)];
    else
        dq_update = [1; 0; 0; 0];
    end
    q_upd = quat_mult(q_upd, dq_update);
    beta_upd = beta_upd + dx(4:6);
end

% =========================================================================
% 3. OUTPUT ASSIGNMENT
% =========================================================================
q_out    = q_upd;
bias_out = beta_upd;
P_out    = P;
w_est    = w_meas - beta_upd;
end

% =========================================================================
% LOCAL FUNCTIONS (Ensuring Mathematical Robustness)
% =========================================================================
function q_res = quat_mult(qA, qB)
    % Hamilton Product: qA ⊗ qB
    % Enforce column vector orientation to prevent cross() function crashes
    wA = qA(1); vA = [qA(2); qA(3); qA(4)];
    wB = qB(1); vB = [qB(2); qB(3); qB(4)];
    
    q_res = [wA*wB - vA'*vB;
             wA*vB + wB*vA + cross(vA, vB)];
             
    q_res = q_res / (norm(q_res) + 1e-12);
end

== matlab function RendezvousSimulator/Navigation Attitude/Star Tracker ==
  settings: updateMethod=DISCRETE  sampleTime=0.01
  data: q_true input; q_meas output
function q_meas = fcn(q_true)

    % Define the sensor accuracy (standard deviation)
    sigma = 9.7e-5;
    
    % Generate a random angular error vector along the 3 axes (white noise)
    % randn is used to sample from a zero-mean Gaussian distribution
    theta_err = sigma * randn(3, 1);
    
    % Convert the small angular error into an error quaternion (dq)
    % Formula: dq = [cos(||theta||/2); sin(||theta||/2) * (theta / ||theta||)]
    mag_err = norm(theta_err);
    if mag_err > 1e-10
        dq = [cos(mag_err/2); (sin(mag_err/2)/mag_err) * theta_err];
    else
        dq = [1; 0; 0; 0];
    end
    
    % Multiply the true quaternion by the error quaternion (Hamilton Product)
    w1 = dq(1); v1 = dq(2:4);
    w2 = q_true(1); v2 = q_true(2:4);
    
    q_meas = [w1*w2 - dot(v1, v2); 
              w1*v2 + w2*v1 + cross(v1, v2)];
          
    % Normalize the measured quaternion to ensure validity
    q_meas = q_meas / norm(q_meas);
end

== matlab function RendezvousSimulator/Position Navigation/Sensor_Manager ==
  data: x_est input; y_meas output; y_gps input; y_lidar input; y_cam input; gps_flag input; sg input; sl_min input; sl_sc input; sc input; R_flat output; update_flag output
function [y_meas, R_flat, update_flag] = Sensor_Manager(x_est, y_gps, y_lidar, y_cam, gps_flag, sg, sl_min, sl_sc, sc)
range = norm(x_est(1:3));
if range > 500
    y_meas=y_gps; sigma=sg; update_flag=double(gps_flag);
elseif range > 30
    y_meas=y_lidar; sigma=max(sl_min,sl_sc*range); update_flag=1;
else
    y_meas=y_cam; sigma=sc; update_flag=1;
end
R_flat=reshape(sigma^2*eye(3),9,1);

== matlab function RendezvousSimulator/Position Navigation/posKF ==
  data: y_meas input; R_flat input; x_out output; a_imu input; dt input; update_flag input; x_in input; P_in input; n input; P_out output
function [x_out, P_out] = posKF(y_meas, R_flat, a_imu, dt, update_flag, x_in, P_in, n)
%% --- State carry-over from previous step ---
x = x_in(:);
P = P_in;
u = a_imu(:);

%% --- Sensor noise ---
sigma_imu = 0.01;     % [m/s^2]  IMU per-axis 1-sigma

%% --- Discrete CW state-transition Phi(dt) and control-input G ---
nt = n*dt; c = cos(nt); s = sin(nt);

Phi_rr = [4-3*c,    0, 0;
          6*(s-nt), 1, 0;
          0,        0, c];
Phi_rv = [ s/n,         2*(1-c)/n,    0;
          -2*(1-c)/n,  (4*s-3*nt)/n,  0;
           0,           0,            s/n];
Phi_vr = [ 3*n*s,     0, 0;
           6*n*(c-1), 0, 0;
           0,         0, -n*s];
Phi_vv = [ c,    2*s,   0;
          -2*s,  4*c-3, 0;
           0,    0,     c];

A = [Phi_rr, Phi_rv;
     Phi_vr, Phi_vv];
B = [0.5*dt^2*eye(3); dt*eye(3)];

%% --- Measurement model: position only ---
H = [eye(3), zeros(3,3)];

%% --- Process noise ---
Q = B*(sigma_imu^2*eye(3))*B';

%% ===== TIME UPDATE (predict) ============================
x_minus = A*x + B*u;
P_minus = A*P*A' + Q;

%% ===== MEASUREMENT UPDATE (correct) ====================
if update_flag > 0.5
    R_meas = reshape(R_flat, 3, 3);
    K = (P_minus*H') / (H*P_minus*H' + R_meas);
    x = x_minus + K*(y_meas(:) - H*x_minus);
    P = (eye(6) - K*H)*P_minus;
    P = 0.5*(P + P');
else
    x = x_minus;
    P = P_minus;
end

x_out = x;
P_out = P;
end

== matlab function RendezvousSimulator/Target/MATLAB Function ==
  data: u input; y output
function y = norm(u)

y = norm(u);

== matlab function RendezvousSimulator/Chaser/MATLAB Function ==
  data: u input; y output
function y = norm(u)

y = norm(u);

== matlab function RendezvousSimulator/MATLAB Function ==
  data: r_c input; r_rel_LVLH output; v_c input; r_t input; v_t input; v_rel_LVLH output; R_ECI2LVLH output
function [r_rel_LVLH, v_rel_LVLH, R_ECI2LVLH] = relative_kinematics(r_c, v_c, r_t, v_t)

    mu = 3.986004418e14;

    r_rel_ECI = r_c - r_t;
    v_rel_ECI = v_c - v_t;
    
    % LVLH Reference basis
    x_hat = r_t/norm(r_t);
    h_vec = cross(r_t, v_t);
    z_hat = h_vec/norm(h_vec);
    y_hat = cross(z_hat, x_hat);
    R_ECI2LVLH = [x_hat'; y_hat'; z_hat'];

    r_rel_LVLH = R_ECI2LVLH*r_rel_ECI;

    n = sqrt(mu / norm(r_t)^3);
    omega = [0; 0; n]; 
    v_rel_LVLH = R_ECI2LVLH*v_rel_ECI - cross(omega, r_rel_LVLH);
end

== matlab function RendezvousSimulator/RCS/Simple RCS/MATLAB Function ==
  data: Tcmd input; u output
function u = control(Tcmd)

      threshold = 2;
      u = zeros(12,1);

      if Tcmd(1) > threshold
          u([9 6 2 11]) = 1;      % +roll
      elseif Tcmd(1) < -threshold
          u([3 12 8 5]) = 1;      % -roll
      end

      if Tcmd(2) > threshold
          u([7 10 3 6]) = 1;      % +pitch
      elseif Tcmd(2) < -threshold
          u([1 4 9 12]) = 1;      % -pitch
      end

      if Tcmd(3) > threshold
          u([1 7 5 11]) = 1;      % +yaw
      elseif Tcmd(3) < -threshold
          u([4 10 2 8]) = 1;      % -yaw
      end

  end

== matlab function RendezvousSimulator/RCS/Simple RCS/MATLAB Function1 ==
  data: t input; Tcmd output
function Tcmd = fcn(t)

    if t < 2
      Tcmd = [5; 0; 0];   % +roll
    elseif t < 4
      Tcmd = [0; 5; 0];   % +pitch
    elseif t < 6
      Tcmd = [0; 0; 5];   % +yaw
    else
      Tcmd = [0; 0; 0];   % off
    end

end

== matlab function RendezvousSimulator/RCS/PWM RCS/MATLAB Function ==
  data: Tcmd input; u output; B input; F input
function u = fcn(Tcmd, B, F)

    u = zeros(12, 1);
    A = [B; F];
    vec = [Tcmd; zeros(3,1)];
    
    u_raw = pinv(A)*vec;
    u_raw(u_raw < 0) = 0; 
   
    max_u = max(u_raw);
    if max_u > 1.0
        u = u_raw/max_u;
    else
        u = u_raw;       
    end
    
end

== matlab function RendezvousSimulator/MATLAB Function2 ==
  data: R input; q output; q_prev input
function q = dcm2quat(R, q_prev)
    
   
    tr = trace(R);
    if tr > 0
        s = 2 * sqrt(1 + tr);
        q_raw = [s/4;
                 (R(3,2) - R(2,3)) / s;
                 (R(1,3) - R(3,1)) / s;
                 (R(2,1) - R(1,2)) / s];
    elseif R(1,1) > R(2,2) && R(1,1) > R(3,3)
        s = 2 * sqrt(1 + R(1,1) - R(2,2) - R(3,3));
        q_raw = [(R(3,2) - R(2,3)) / s;
                 s/4;
                 (R(1,2) + R(2,1)) / s;
                 (R(1,3) + R(3,1)) / s];
    elseif R(2,2) > R(3,3)
        s = 2 * sqrt(1 + R(2,2) - R(1,1) - R(3,3));
        q_raw = [(R(1,3) - R(3,1)) / s;
                 (R(1,2) + R(2,1)) / s;
                 s/4;
                 (R(2,3) + R(3,2)) / s];
    else
        s = 2 * sqrt(1 + R(3,3) - R(1,1) - R(2,2));
        q_raw = [(R(2,1) - R(1,2)) / s;
                 (R(1,3) + R(3,1)) / s;
                 (R(2,3) + R(3,2)) / s;
                 s/4];
    end
    
    q_raw = q_raw / norm(q_raw);

    
    if (q_raw' * q_prev) < 0
        q = -q_raw; 
    else
        q = q_raw;  
    end
end

== matlab function RendezvousSimulator/RCS/PWM RCS/MATLAB Function1 ==
  data: u_req input; u_cmd output; t input; T_cycle input; MIB input
function u_cmd = rcs_pwm_mapper(u_req, t, T_cycle, MIB)
    % Inputs:
    % u_req   : 12x1 array of commanded duty cycles (values from 0.0 to 1.0)
    % t       : Current simulation clock time (seconds)
    % T_cycle : Total duration of one control cycle (e.g., 0.1 seconds)
    % MIB     : Minimum Impulse Bit threshold (e.g., 0.05 seconds)
    
    % Output:
    % u_cmd   : 12x1 array of discrete 0 or 1 commands for the valves

    % Initialize the output vector with all valves closed
    u_cmd = zeros(12, 1);

    % Find our current position within the repeating control cycle
    t_current = mod(t, T_cycle);

    % Evaluate all 12 thrusters
    for i = 1:12
        
        % Calculate how many seconds this specific valve is asked to open
        t_on_requested = u_req(i)*T_cycle;
        
        % THE DEADBAND: Check against the physical MIB limit
        if t_on_requested < MIB
            % If the request is too short, throw it away
            t_on_actual = 0; 
        else
            % If it is a physically valid request, approve it
            t_on_actual = t_on_requested; 
        end
        
        % THE PWM LOGIC: Open or close the valve based on the clock
        if t_current <= t_on_actual
            u_cmd(i) = 1;  % Energize valve (ON)
        else
            u_cmd(i) = 0;  % De-energize valve (OFF)
        end
        
    end
end

== matlab function RendezvousSimulator/Position Navigation/LIDAR_Sigma ==
  data: x_est input; sigma output; sig_min input; sig_scale input
function sigma = LIDAR_Sigma(x_est, sig_min, sig_scale)
sigma = max(sig_min, sig_scale * norm(x_est(1:3)));
